simulink model "p7dinamico"  (R2017b)
settings: Solver=VariableStepAuto  StartTime=0.0  StopTime=10  MinStep=0.001  RelTol=1e-3
libraries: simulink x1
settings Model: Creator=Rita Monteiro  LastModifiedBy=Rita Monteiro

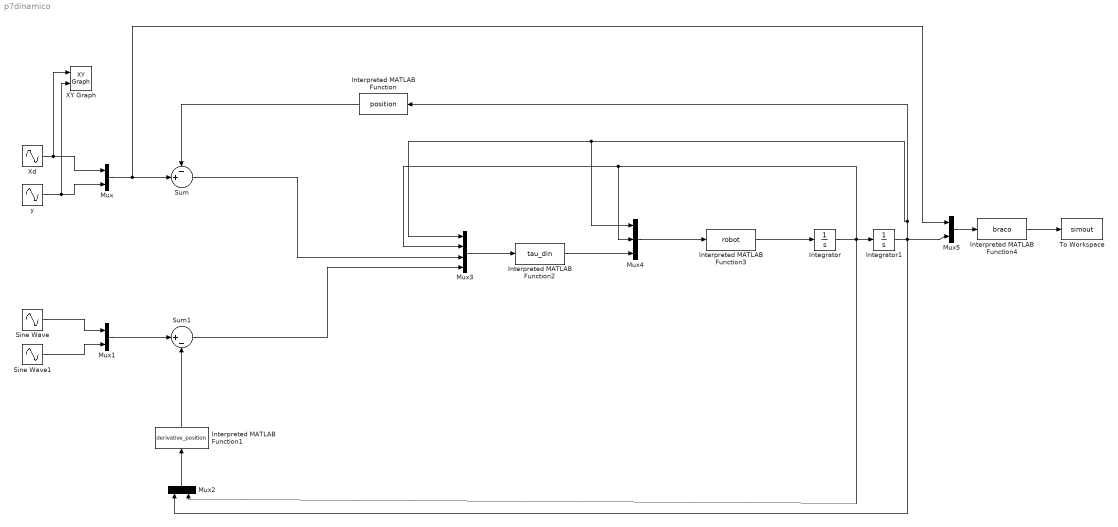
== system p7dinamico ==
  Integrator : Integrator  InitialCondition=[0;0]
  Integrator1 : Integrator  InitialCondition=[pi/2;-pi/4]
  Interpreted MATLAB Function : MATLABFcn  MATLABFcn=position
  Interpreted MATLAB Function1 : MATLABFcn  MATLABFcn=derivative_position
  Interpreted MATLAB Function2 : MATLABFcn  MATLABFcn=tau_din
  Interpreted MATLAB Function3 : MATLABFcn  MATLABFcn=robot
  Interpreted MATLAB Function4 : MATLABFcn  MATLABFcn=braco  OutputDimensions=1
  Mux{,1..2,5} (4 alike) : Mux  Inputs=2
  Mux3 : Mux
  Mux4 : Mux  Inputs=3
  Sine Wave : Sin  Amplitude=0.12*(2*pi*0.25)  Frequency=2*pi*0.25  Phase=pi  SampleTime=0
  Sine Wave1 : Sin  Amplitude=0.07*(2*pi*0.25)  Frequency=2*pi*0.25  Phase=pi/2  SampleTime=0
  Sum : Sum  Inputs=-+|
  Sum1 : Sum  Inputs=|+-
  To Workspace : ToWorkspace  VariableName=simout  SaveFormat=Timeseries  SampleTime=-1
  XY Graph : simulink/Sinks/XY Graph  xmin=-1  xmax=1  ymin=-1  ymax=1  st=-1
  Xd : Sin  Amplitude=0.12  Bias=0.25  Frequency=2*pi*(1/4)  Phase=pi/2  SampleTime=0
  y : Sin  Amplitude=0.07  Bias=0.2  Frequency=2*pi*(1/4)  SampleTime=0
  wires:
  y/1 -> XY Graph/2, Mux/2
  Xd/1 -> XY Graph/1, Mux/1
  Sine Wave1/1 -> Mux1/2
  Sine Wave/1 -> Mux1/1
  Mux/1 -> Mux5/1, Sum/2
  Interpreted MATLAB Function/1 -> Sum/1
  Mux1/1 -> Sum1/1
  Interpreted MATLAB Function1/1 -> Sum1/2
  Mux2/1 -> Interpreted MATLAB Function1/1
  Sum1/1 -> Mux3/4
  Mux3/1 -> Interpreted MATLAB Function2/1
  Interpreted MATLAB Function2/1 -> Mux4/3
  Mux4/1 -> Interpreted MATLAB Function3/1
  Interpreted MATLAB Function3/1 -> Integrator/1
  Integrator/1 -> Mux4/2, Mux3/2, Integrator1/1, Mux2/2
  Integrator1/1 -> Mux4/1, Mux3/1, Interpreted MATLAB Function/1, Mux5/2, Mux2/1
  Mux5/1 -> Interpreted MATLAB Function4/1
  Interpreted MATLAB Function4/1 -> To Workspace/1
  Sum/1 -> Mux3/3
